simulink model "model"  (R2016a)
settings: Solver=ode4  StartTime=0.0  StopTime=60  FixedStep=0.001  RelTol=1e-3
values from neighbouring files (symbols this model uses):
  D1 = par(2)    [cel.m]    (also in cel_P.m; cel_PD2.m = 38.2416; dane.m; dane.mat = 35.0184631454)
  D2 = par(4)    [cel.m]    (also in cel_P.m; cel_PD2.m = par(2); cel_z.m = par(2); dane.m)
  I3 = par(6)    [cel.m]    (also in cel_PD2.m = 0.0358; cel_bezFeedforward.m = par(2); dane.m; dane.mat = 0.0341130667622)
  Ko = 10    [dane.m]    (also in dane.mat; dane2.mat; dane3.mat; dane4.mat)
  Kr = par(7)    [cel.m]    (also in cel_P.m = par(5); cel_PD2.m = 0.3949; cel_bezFeedforward.m = par(3); dane.m)
  Kw1 = 10    [dane.m]    (also in dane.mat; dane2.mat; dane3.mat; dane4.mat)
  Kw2 = 5    [dane.m]    (also in dane.mat; dane2.mat; dane3.mat; dane4.mat)
  limit2 = 40    [dane.m]    (also in dane.mat; dane2.mat; dane3.mat; dane4.mat)
  limit3 = 40    [dane.m]    (also in dane.mat; dane2.mat; dane3.mat; dane4.mat)
  P1 = par(1)    [cel.m]    (also in cel_P.m; cel_PD2.m = 0.0302; dane.m; dane.mat = 0.804768322622)
  P2 = par(3)    [cel.m]    (also in cel_P.m; cel_PD2.m = par(1); cel_z.m = par(1); dane.m)
  P3 = par(5)    [cel.m]    (also in cel_PD2.m = 6.71669750093e-06; cel_bezFeedforward.m = par(1); dane.m; dane.mat = 3.3559799843e-06)
  r = zad(index)    [dane.m]    (also in dane.mat = 50; dane2.mat = 20; dane3.mat = 70; dane4.mat = 70)
  tau = 1    [dane.m]    (also in dane.mat; dane2.mat; dane3.mat; dane4.mat)
  To = 1    [dane.m]    (also in dane.mat; dane2.mat; dane3.mat; dane4.mat)
  Tw2 = .1    (= 0.1)    [dane.m]    (also in dane.mat; dane2.mat; dane3.mat; dane4.mat)
  z1 = 0    [dane.m]    (also in dane.mat; optymalizacja.m; optymalizacja_bezFeedforward.m; optymalizacja_new.m)
libraries: simulink x2
settings Model: Creator=Maciek  LastModifiedBy=Maciek
settings GRTTargetCC: GeneratePreprocessorConditionals=Use local settings

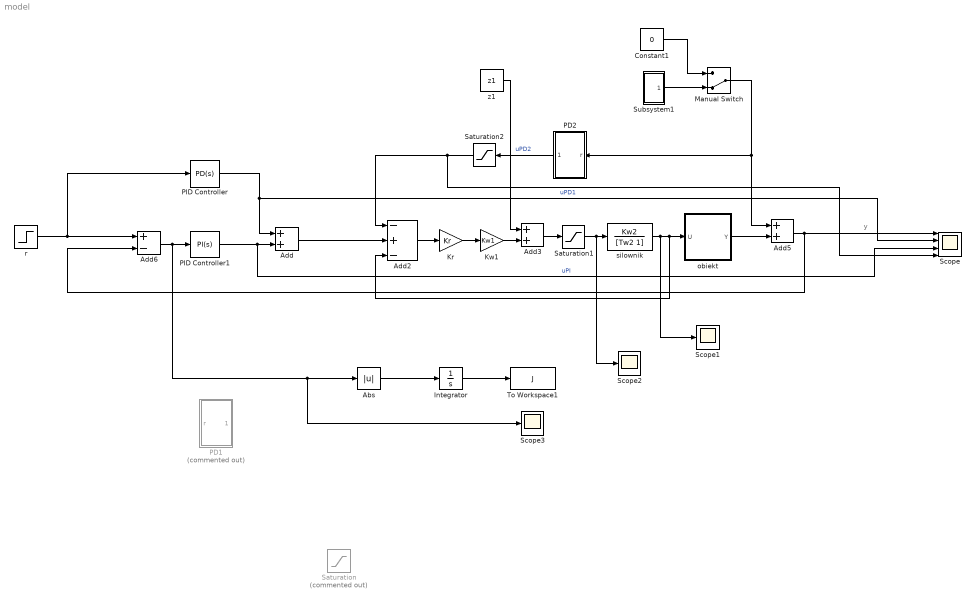
== system model ==
  note: y
  Abs : Abs
  Add : Sum
  Add2 : Sum  Inputs=-+-
  Add3 : Sum
  Add5 : Sum
  Add6 : Sum  Inputs=+-
  Constant1 : Constant  Value=0
  Integrator : Integrator
  Kr : Gain  Gain=Kr
  "Kw1 " : Gain  Gain=Kw1
  Manual Switch : ManualSwitch  CurrentSetting=0
  PD1 : Subsystem  Commented=on
  PD2 : Subsystem
  PID Controller : simulink/Continuous/PID Controller  Controller=PD  TimeDomain=Continuous-time  SampleTime=-1  IntegratorMethod=Forward Euler  FilterMethod=Forward Euler  Form=Parallel  UseFilter=on  ControllerParametersSource=internal  P=P1  I=1  D=D1  N=100  InitialConditionSource=internal  InitialConditionForIntegrator=0  InitialConditionForFilter=0  ExternalReset=none  LimitOutput=on  UpperSaturationLimit=inf  LowerSaturationLimit=-inf  LinearizeAsGain=on  AntiWindupMode=none  Kb=1  TrackingMode=off  Kt=1  PParamMin=[]  PParamMax=[]  IParamMin=[]  IParamMax=[]  DParamMin=[]  DParamMax=[]  NParamMin=[]  NParamMax=[]  KbParamMin=[]  KbParamMax=[]  KtParamMin=[]  KtParamMax=[]  POutMin=[]  POutMax=[]  IOutMin=[]  IOutMax=[]  DOutMin=[]  DOutMax=[]  NOutMin=[]  NOutMax=[]  KbOutMin=[]  KbOutMax=[]  KtOutMin=[]  KtOutMax=[]  IntegratorOutMin=[]  IntegratorOutMax=[]  FilterOutMin=[]  FilterOutMax=[]  SumOutMin=[]  SumOutMax=[]  SumI1OutMin=[]  SumI1OutMax=[]  SumI2OutMin=[]  SumI2OutMax=[]  SumI3OutMin=[]  SumI3OutMax=[]  SumDOutMin=[]  SumDOutMax=[]  SaturationOutMin=[]  SaturationOutMax=[]  IntegratorContinuousStateAttributes=''  IntegratorStateMustResolveToSignalObject=off  IntegratorRTWStateStorageClass=Auto  FilterContinuousStateAttributes=''  FilterStateMustResolveToSignalObject=off  FilterRTWStateStorageClass=Auto  DifferentiatorICPrevScaledInput=0  DifferentiatorOutMin=[]  DifferentiatorOutMax=[]
  PID Controller1 : simulink/Continuous/PID Controller  Controller=PI  TimeDomain=Continuous-time  SampleTime=-1  IntegratorMethod=Forward Euler  FilterMethod=Forward Euler  Form=Parallel  UseFilter=on  ControllerParametersSource=internal  P=P3  I=I3  D=0  N=100  InitialConditionSource=internal  InitialConditionForIntegrator=0  InitialConditionForFilter=0  ExternalReset=none  LimitOutput=on  UpperSaturationLimit=inf  LowerSaturationLimit=-inf  LinearizeAsGain=on  AntiWindupMode=back-calculation  Kb=1/sqrt(max(0.001,I3))  TrackingMode=off  Kt=1  PParamMin=[]  PParamMax=[]  IParamMin=[]  IParamMax=[]  DParamMin=[]  DParamMax=[]  NParamMin=[]  NParamMax=[]  KbParamMin=[]  KbParamMax=[]  KtParamMin=[]  KtParamMax=[]  POutMin=[]  POutMax=[]  IOutMin=[]  IOutMax=[]  DOutMin=[]  DOutMax=[]  NOutMin=[]  NOutMax=[]  KbOutMin=[]  KbOutMax=[]  KtOutMin=[]  KtOutMax=[]  IntegratorOutMin=[]  IntegratorOutMax=[]  FilterOutMin=[]  FilterOutMax=[]  SumOutMin=[]  SumOutMax=[]  SumI1OutMin=[]  SumI1OutMax=[]  SumI2OutMin=[]  SumI2OutMax=[]  SumI3OutMin=[]  SumI3OutMax=[]  SumDOutMin=[]  SumDOutMax=[]  SaturationOutMin=[]  SaturationOutMax=[]  IntegratorContinuousStateAttributes=''  IntegratorStateMustResolveToSignalObject=off  IntegratorRTWStateStorageClass=Auto  FilterContinuousStateAttributes=''  FilterStateMustResolveToSignalObject=off  FilterRTWStateStorageClass=Auto  DifferentiatorICPrevScaledInput=0  DifferentiatorOutMin=[]  DifferentiatorOutMax=[]
  Saturation : Saturate  Commented=on  UpperLimit=limit3  LowerLimit=-limit3
  Saturation1 : Saturate  UpperLimit=limit2  LowerLimit=-limit2
  Saturation2 : Saturate  UpperLimit=limit2  LowerLimit=-limit2
  Scope : Scope  NumInputPorts=4
  Scope1 : Scope
  Scope2 : Scope
  Scope3 : Scope
  Subsystem1 : Subsystem
  To Workspace1 : ToWorkspace  VariableName=J  SampleTime=-1
      settings: MaxDataPoints=1
  obiekt : Subsystem
  r : Step  After=r  SampleTime=0
  silownik : TransferFcn  Numerator=Kw2  Denominator=[Tw2 1]
  z1 : Constant  Value=z1
  wires:
  r/1 -> PID Controller/1, Add6/1
  PID Controller/1 -> Add/1, Scope/2  "uPD1"
  Kr/1 -> "Kw1 "/1
  "Kw1 "/1 -> Add3/2
  Add3/1 -> Saturation1/1
  z1/1 -> Add3/1
  PID Controller1/1 -> Add/2, Scope/3  "uPI"
  Add6/1 -> PID Controller1/1, Scope3/1, Abs/1
  Manual Switch/1 -> PD2/1(r), Add5/1
  Add5/1 -> Scope/1, Add6/2
  PD2/1(uPD2) -> Saturation2/1  "uPD2"
  obiekt/1(Y) -> Add5/2
  Add2/1 -> Kr/1
  silownik/1 -> Scope1/1, Add2/3, obiekt/1(U)
  Integrator/1 -> To Workspace1/1
  Abs/1 -> Integrator/1
  Subsystem1/1(Out1) -> Manual Switch/2
  Constant1/1 -> Manual Switch/1
  Add/1 -> Add2/2
  Saturation1/1 -> Scope2/1, silownik/1
  Saturation2/1 -> Scope/4, Add2/1

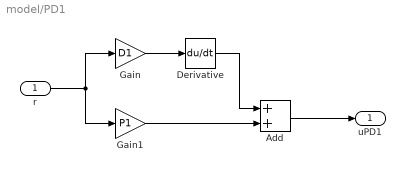
== system model/PD1 ==
  r : Inport
  Add : Sum
  Derivative : Derivative
  Gain : Gain  Gain=D1
  Gain1 : Gain  Gain=P1
  uPD1 : Outport
  wires:
  Derivative/1 -> Add/1
  Gain1/1 -> Add/2
  r/1 -> Gain/1, Gain1/1
  Gain/1 -> Derivative/1
  Add/1 -> uPD1/1

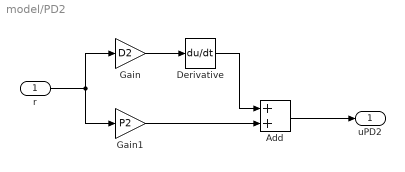
== system model/PD2 ==
  r : Inport
  Add : Sum
  Derivative : Derivative
  Gain : Gain  Gain=D2
  Gain1 : Gain  Gain=P2
  uPD2 : Outport
  wires:
  Derivative/1 -> Add/1
  Gain1/1 -> Add/2
  r/1 -> Gain/1, Gain1/1
  Gain/1 -> Derivative/1
  Add/1 -> uPD2/1

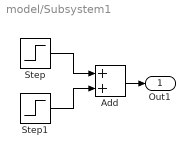
== system model/Subsystem1 ==
  Add : Sum
  Step : Step  Time=20  After=5  SampleTime=0
  Step1 : Step  Time=25  After=-5  SampleTime=0
  Out1 : Outport
  wires:
  Add/1 -> Out1/1
  Step/1 -> Add/1
  Step1/1 -> Add/2

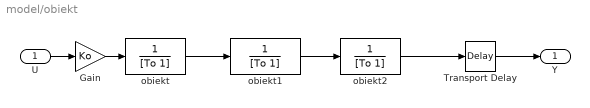
== system model/obiekt ==
  U : Inport
  Gain : Gain  Gain=Ko
  Transport Delay : TransportDelay  DelayTime=tau
  obiekt : TransferFcn  Numerator=1  Denominator=[To 1]
  obiekt1 : TransferFcn  Numerator=1  Denominator=[To 1]
  obiekt2 : TransferFcn  Numerator=1  Denominator=[To 1]
  Y : Outport
  wires:
  U/1 -> Gain/1
  Gain/1 -> obiekt/1
  obiekt/1 -> obiekt1/1
  obiekt1/1 -> obiekt2/1
  Transport Delay/1 -> Y/1
  obiekt2/1 -> Transport Delay/1
